simulink model "Copy_of_AB_Final_of_MPC_Bandwidth_Result"  (R2022b)
settings: Solver=FixedStepDiscrete  StartTime=0.0  StopTime=Inf  FixedStep=100e-6  RelTol=1e-3  EnableMultiTasking=on
undefined symbols (not defined in the file): C28x, CPU1, CPU2, CurrentBypassValue, DiscIntNeverNeededParam, Down, GPTRIP1SEL, TZ1, Up
libraries: c2802xlib x31, simulink x22, dspstat3 x17, dspsigops x9, c2837xDlib x6, c280xlib x5, PID_Lib x2, c2000lib x1, spsAlphaBetaZerotoabcLib x1, spsAlphaBetaZerotodq0Lib x1
(part 1 of 8)
settings Model: ExtModeTrigDuration=8  Creator=user  LastModifiedBy=user
settings SolverCC: AutoInsertRateTranBlk=on
settings OptimizationCC: DefaultParameterBehavior=Inlined  DefaultUnderspecifiedDataType=single  EnhancedBackFolding=on  PassReuseOutputArgsAs=Individual arguments  MaxStackSize=1024  OptimizeBlockOrder=speed  DifferentSizesBufferReuse=on  OptimizationCustomize=off  DenormalBehavior=FlushToZero  EfficientTunableParamExpr=on
settings DebuggingCC: ParameterTunabilityLossMsg=error
settings HardwareCC: ProdBitPerChar=16  ProdBitPerInt=16  ProdBitPerPointer=32  ProdBitPerSizeT=32  ProdBitPerPtrDiffT=32  ProdLargestAtomicInteger=Integer  ProdLargestAtomicFloat=None  ProdWordSize=16  ProdLongLongMode=on  ProdHWDeviceType=Texas Instruments->C2000
settings ModelReferenceCC: ModelReferenceNumInstancesAllowed=Single
settings SFSimCC: MATLABDynamicMemAlloc=off
settings RTWCC: Description=Embedded Coder  SystemTargetFile=ert.tlc  HardwareBoard=TI Delfino F28379D LaunchPad  TLCOptions=-aInlineSetEventsForThisBaseRateFcn=TLC_FALSE -aSuppressMultiTaskScheduler=TLC_FALSE -aRateBasedStepFcn=1  TemplateMakefile=ert_default_tmf  GenerateReport=on  Toolchain=Texas Instruments Code Composer Studio (C2000)  LaunchReport=on
settings CodeAppCC: ForceParamTrailComments=on  IgnoreCustomStorageClasses=off  OperatorAnnotations=on  SimulinkDataObjDesc=on  SFDataObjDesc=on  InsertBlockDesc=on
settings ERTTargetCC: CodeReplacementLibrary=TI C28x  ExtModeTransport=4  ExtModeStaticAlloc=on  ExtModeAutomaticAllocSize=off  ExtModeStaticAllocSize=10000  ExtModeMexFile=ext_xcp  ExtModeIntrfLevel=Level2 - Open  InlinedParameterPlacement=NonHierarchical

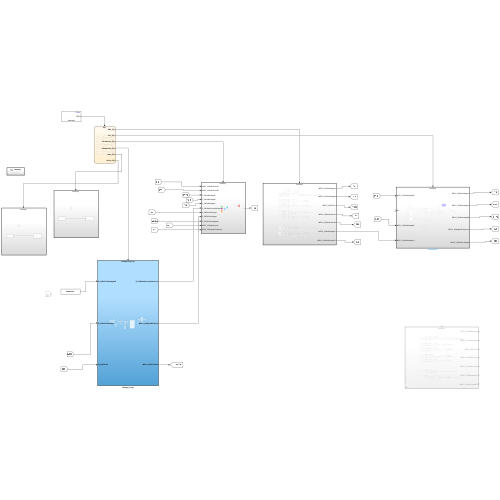
[thumbnail: Simulink's stored preview of the top-level diagram]
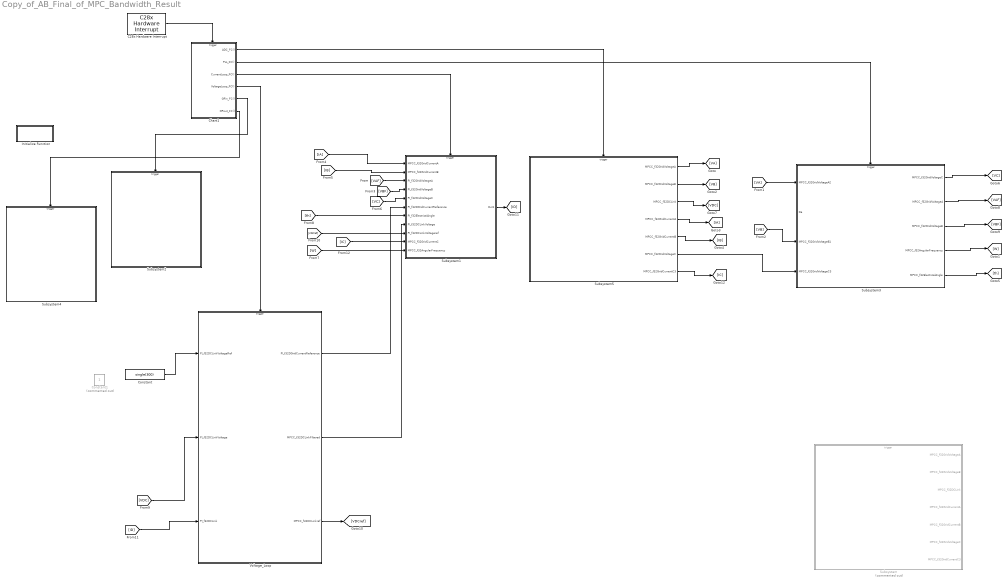
== system Copy_of_AB_Final_of_MPC_Bandwidth_Result ==
  C28x Hardware Interrupt : c2000lib/Scheduling/C28x Hardware Interrupt  irqnumbers=[1]  pienumbers=[1]  irqpriorities=[1]  irqpreempts=[0]  showinput=off  dspchiptype=C280X
  Chart1 : Stateflow chart  TreatAsAtomicUnit=on
  Constant : Constant  Value=single(300)
  Constant1 : Constant  Commented=on
  Initialize Function : Subsystem  TreatAsAtomicUnit=on
  Subsystem : Subsystem  Commented=on
  Subsystem1 : Subsystem
  Subsystem2 : Subsystem
  Subsystem3 : Subsystem
  Subsystem4 : Subsystem
  Subsystem5 : Subsystem
  Voltage_Loop : Subsystem
  wires:
  Chart1/5(GPin_FC()) -> Subsystem2/Trigger
  Chart1/3(CurrentLoop_FC()) -> Subsystem1/Trigger
  Chart1/4(VoltageLoop_FC()) -> Voltage_Loop/Trigger
  C28x Hardware Interrupt/1 -> Chart1/Trigger
  Chart1/6(GPout_FC()) -> Subsystem4/Trigger
  Chart1/2(PLL_FC()) -> Subsystem3/Trigger
  Chart1/1(ADC_FC()) -> Subsystem5/Trigger
  [IA] -> Subsystem1/1(MPCC_f32GridCurrentA)
  [IB] -> Subsystem1/2(MPCC_f32GridCurrentB)
  Subsystem3/1(MPCC_f32GridVoltageC) -> [VC]
  [th] -> Subsystem1/7(PI_f32ElectricalAngle)
  Voltage_Loop/2(MPCC_f32DCLinkFiltered) -> Subsystem1/8(PI_f32DCLinkVoltage)
  Voltage_Loop/1(PI_f32DGridCurrentReference) -> Subsystem1/6(PI_f32DGridCurrentReference)
  [VA] -> Subsystem3/1(MPCC_f32GridVoltageA2)
  [VAF] -> Subsystem1/3(PI_f32GridVoltageA)
  [VC] -> Subsystem1/5(PI_f32GridVoltageC)
  [VBF] -> Subsystem1/4(PI_f32GridVoltageB)
  Subsystem3/2(MPCC_f32GridVoltageA) -> [VAF]
  Subsystem3/3(MPCC_f32GridVoltageB) -> [VBF]
  Voltage_Loop/3(MPCC_f32DCLinkref) -> [VDCref]
  [VDCref] -> Subsystem1/9(PI_f32DCLinkVoltageref)
  [VDC] -> Voltage_Loop/2(PI_f32DCLinkVoltage)
  Constant/1 -> Voltage_Loop/1(PI_f32DCLinkVoltageRef)
  [VB] -> Subsystem3/3(MPCC_f32GridVoltageB1)
  Subsystem1/1(Out1) -> [ID]
  [ID] -> Voltage_Loop/3(PI_f32DCLink)
  [IC] -> Subsystem1/10(MPCC_f32GridCurrentC)
  [W] -> Subsystem1/11(MPCC_f32AngularFrequency)
  Subsystem3/4(MPCC_f32AngularFrequency) -> [W]
  Subsystem3/5(MPCC_f32ElectricalAngle) -> [th]
  Subsystem5/2(MPCC_f32GridVoltageB) -> [VB]
  Subsystem5/1(MPCC_f32GridVoltageA) -> [VA]
  Subsystem5/3(MPCC_f32DCLink) -> [VDC]
  Subsystem5/4(MPCC_f32GridCurrentA) -> [IA]
  Subsystem5/5(MPCC_f32GridCurrentB) -> [IB]
  Subsystem5/7(MPCC_f32GridCurrentC3) -> [IC]
  Subsystem5/6(MPCC_f32GridVoltageC) -> Subsystem3/4(MPCC_f32GridVoltageC3)

== system Copy_of_AB_Final_of_MPC_Bandwidth_Result/Initialize Function ==
  Constant : Constant  Value=boolean(0)
  Digital Output : c2837xDlib/Digital Output  GPIO_Number=GPIO8~GPIO15  GPIO_Bit0=off  GPIO_BIT0_Toggle=off  GPIO_Bit1=off  GPIO_BIT1_Toggle=off  GPIO_Bit2=off  GPIO_BIT2_Toggle=off  GPIO_Bit3=on  GPIO_BIT3_Toggle=off  GPIO_Bit4=off  GPIO_BIT4_Toggle=off  GPIO_Bit5=off  GPIO_BIT5_Toggle=off  GPIO_Bit6=off  GPIO_BIT6_Toggle=off  GPIO_Bit7=off  GPIO_BIT7_Toggle=off
  Event Listener : EventListener  DisableCoverage=on  EventName=reset
  wires:
  Constant/1 -> Digital Output/1

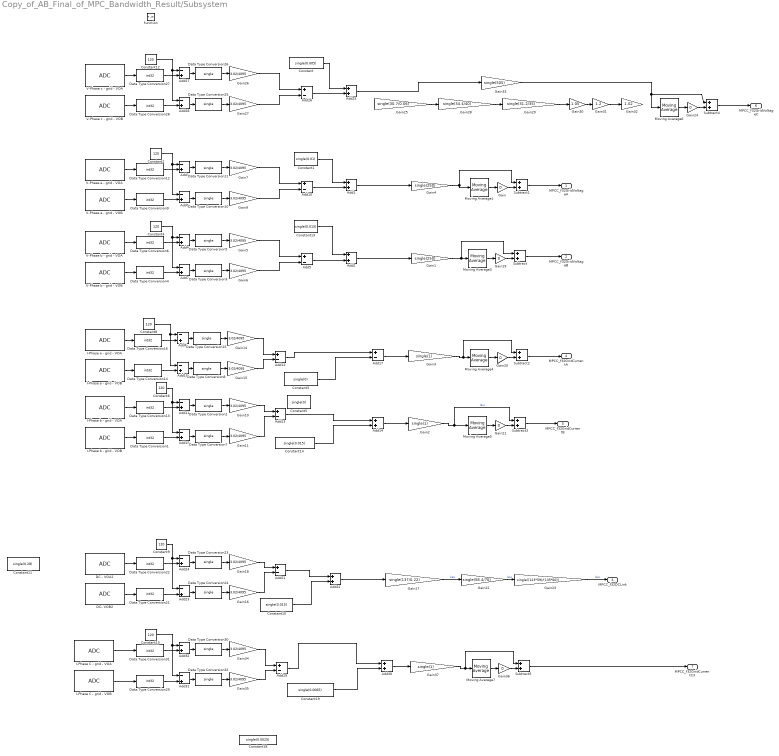
== system Copy_of_AB_Final_of_MPC_Bandwidth_Result/Subsystem ==
  function : TriggerPort  TriggerType=function-call  VariantControl=(inherit)
  Add{1..2,14,22,25,30} (6 alike) : Sum  AccumDataTypeStr=single  OutDataTypeStr=single
  Add{5,10,12..13,17,21,26,29} (8 alike) : Sum  Inputs=+-  AccumDataTypeStr=single  OutDataTypeStr=single
  Add{3..4,6..7,9,11,15,18,23..24,27..28,31..32} (14 alike) : Sum  Inputs=-+  AccumDataTypeStr=single  OutDataTypeStr=single
  Constant : Constant  Value=single(0.005)
  Constant1 : Constant  Value=single(0.01)
  Constant10 : Constant  Value=single(0.015)
  Constant11 : Constant  Value=single(0.28)
  Constant{2,4,6,8..9,12,15} (7 alike) : Constant  Value=120  OutDataTypeStr=single
  Constant13 : Constant  Value=single(0.015)
  Constant14 : Constant  Value=single(0.015)
  Constant18 : Constant  Value=single(0.0025)
  Constant19 : Constant  Value=single(0.0065)
  Constant3 : Constant  Value=single(0)
  Constant5 : Constant  Value=single(0)
  DC - VOA2 : c2802xlib/ADC  blkParamProc=C2000_Type4  ADCModule=C  samplingMode=Single sample mode  ADCResolution=12-bit (Single-ended input)  useSOC1=SOC0  useSOC2=SOC0_SOC1  SOCAcquisitionWindow=22  SOCTriggerSource=ePWM1_ADCSOCA  SOCInterruptTrigger=No ADCINT  Ts=-1  dType=uint16  postInterrupt=off  interruptSel=ADCINT1  ADCINTContinuous=on  endma=off  chdma=1  conv1=ADCINA0  conv2=ADCINA0 and ADCINB0  conv1_Type4=ADCIN5  conv2_Type4=ADCIN0 and ADCIN1
  DC- VOB2 : c2802xlib/ADC  blkParamProc=C2000_Type4  ADCModule=B  samplingMode=Single sample mode  ADCResolution=12-bit (Single-ended input)  useSOC1=SOC3  useSOC2=SOC0_SOC1  SOCAcquisitionWindow=22  SOCTriggerSource=ePWM1_ADCSOCA  SOCInterruptTrigger=No ADCINT  Ts=-1  dType=uint16  postInterrupt=off  interruptSel=ADCINT2  ADCINTContinuous=on  endma=off  chdma=1  conv1=ADCINA0  conv2=ADCINA0 and ADCINB0  conv1_Type4=ADCIN5  conv2_Type4=ADCIN2 and ADCIN3
  Data Type Conversion{1,4,6,9,12..14,16,21..22,27..29,31} (14 alike) : DataTypeConversion  OutDataTypeStr=int32  ConvertRealWorld=Stored Integer (SI)  SaturateOnIntegerOverflow=off  RndMeth=Floor
  Data Type Conversion{2..3,5,7..8,10..11,15,23..26,30,32} (14 alike) : DataTypeConversion  OutDataTypeStr=single  SaturateOnIntegerOverflow=off  RndMeth=Floor
  Gain{,19..21,24,36} (6 alike) : Gain  Gain=0
  Gain1 : Gain  Gain=single(250)
  Gain{5..7,9..11,14..16,18,26..27,34..35} (14 alike) : Gain  Gain=3.02/4095  ParamDataTypeStr=single  OutDataTypeStr=single
  Gain17 : Gain  Gain=single(137/0.22)
  Gain2 : Gain  Gain=single(1)
  Gain22 : Gain  Gain=single(58.4/70)
  Gain23 : Gain  Gain=single((123*59)/(135*60))
  Gain25 : Gain  Gain=single(30.7/0.06)
  Gain28 : Gain  Gain=single(34.4/40)
  Gain29 : Gain  Gain=single(31.2/35)
  Gain3 : Gain  Gain=single(1)
  Gain30 : Gain  Gain=1.05
  Gain31 : Gain  Gain=1.2
  Gain32 : Gain  Gain=1.02
  Gain33 : Gain  Gain=single(505)
  Gain37 : Gain  Gain=single(1)
  Gain4 : Gain  Gain=single(250)
  I-Phase C - grid - VOA : c2802xlib/ADC  blkParamProc=C2000_Type4  ADCModule=A  samplingMode=Single sample mode  ADCResolution=12-bit (Single-ended input)  useSOC1=SOC15  useSOC2=SOC0_SOC1  SOCAcquisitionWindow=22  SOCTriggerSource=ePWM1_ADCSOCA  SOCInterruptTrigger=No ADCINT  Ts=-1  dType=uint16  postInterrupt=off  interruptSel=ADCINT1  ADCINTContinuous=on  endma=off  chdma=1  conv1=ADCINA0  conv2=ADCINA0 and ADCINB0  conv1_Type4=ADCIN15  conv2_Type4=ADCIN0 and ADCIN1
  I-Phase C - grid - VOB : c2802xlib/ADC  blkParamProc=C2000_Type4  ADCModule=A  samplingMode=Single sample mode  ADCResolution=12-bit (Single-ended input)  useSOC1=SOC10  useSOC2=SOC0_SOC1  SOCAcquisitionWindow=22  SOCTriggerSource=ePWM1_ADCSOCA  SOCInterruptTrigger=No ADCINT  Ts=-1  dType=uint16  postInterrupt=off  interruptSel=ADCINT2  ADCINTContinuous=on  endma=off  chdma=1  conv1=ADCINA0  conv2=ADCINA0 and ADCINB0  conv1_Type4=ADCIN14  conv2_Type4=ADCIN2 and ADCIN3
  I-Phase a - grid - VOA : c2802xlib/ADC  blkParamProc=C2000_Type4  ADCModule=A  samplingMode=Single sample mode  ADCResolution=12-bit (Single-ended input)  useSOC1=SOC0  useSOC2=SOC0_SOC1  SOCAcquisitionWindow=22  SOCTriggerSource=ePWM1_ADCSOCA  SOCInterruptTrigger=No ADCINT  Ts=-1  dType=uint16  postInterrupt=on  interruptSel=ADCINT1  ADCINTContinuous=on  endma=off  chdma=1  conv1=ADCINA0  conv2=ADCINA0 and ADCINB0  conv1_Type4=ADCIN4  conv2_Type4=ADCIN0 and ADCIN1
  I-Phase a - grid - VOB : c2802xlib/ADC  blkParamProc=C2000_Type4  ADCModule=B  samplingMode=Single sample mode  ADCResolution=12-bit (Single-ended input)  useSOC1=SOC1  useSOC2=SOC0_SOC1  SOCAcquisitionWindow=22  SOCTriggerSource=ePWM1_ADCSOCA  SOCInterruptTrigger=No ADCINT  Ts=-1  dType=uint16  postInterrupt=off  interruptSel=ADCINT2  ADCINTContinuous=on  endma=off  chdma=1  conv1=ADCINA0  conv2=ADCINA0 and ADCINB0  conv1_Type4=ADCIN4  conv2_Type4=ADCIN2 and ADCIN3
  I-Phase b - grid - VOA : c2802xlib/ADC  blkParamProc=C2000_Type4  ADCModule=C  samplingMode=Single sample mode  ADCResolution=12-bit (Single-ended input)  useSOC1=SOC12  useSOC2=SOC0_SOC1  SOCAcquisitionWindow=22  SOCTriggerSource=ePWM1_ADCSOCA  SOCInterruptTrigger=No ADCINT  Ts=-1  dType=uint16  postInterrupt=off  interruptSel=ADCINT1  ADCINTContinuous=on  endma=off  chdma=1  conv1=ADCINA0  conv2=ADCINA0 and ADCINB0  conv1_Type4=ADCIN4  conv2_Type4=ADCIN0 and ADCIN1
  I-Phase b - grid - VOB : c2802xlib/ADC  blkParamProc=C2000_Type4  ADCModule=A  samplingMode=Single sample mode  ADCResolution=12-bit (Single-ended input)  useSOC1=SOC3  useSOC2=SOC0_SOC1  SOCAcquisitionWindow=22  SOCTriggerSource=ePWM1_ADCSOCA  SOCInterruptTrigger=No ADCINT  Ts=-1  dType=uint16  postInterrupt=off  interruptSel=ADCINT2  ADCINTContinuous=on  endma=off  chdma=1  conv1=ADCINA0  conv2=ADCINA0 and ADCINB0  conv1_Type4=ADCIN5  conv2_Type4=ADCIN2 and ADCIN3
  Moving Average{1,3..7} (6 alike) : dspstat3/Moving Average  Method=Exponential weighting  ForgettingFactorPort=off  SpecifyWindowLength=on  WindowLength=4  OverlapLength=3  AllowArbitraryInputLength=off  ForgettingFactor=0.99  SimulateUsing=Code generation
  Subtract{,1..5} (6 alike) : Sum
  V-Phase a - grid - VOA : c2802xlib/ADC  blkParamProc=C2000_Type4  ADCModule=C  samplingMode=Single sample mode  ADCResolution=12-bit (Single-ended input)  useSOC1=SOC4  useSOC2=SOC0_SOC1  SOCAcquisitionWindow=22  SOCTriggerSource=ePWM1_ADCSOCA  SOCInterruptTrigger=No ADCINT  Ts=-1  dType=uint16  postInterrupt=off  interruptSel=ADCINT1  ADCINTContinuous=on  endma=off  chdma=1  conv1=ADCINA0  conv2=ADCINA0 and ADCINB0  conv1_Type4=ADCIN3  conv2_Type4=ADCIN0 and ADCIN1
  V-Phase a - grid - VOB : c2802xlib/ADC  blkParamProc=C2000_Type4  ADCModule=B  samplingMode=Single sample mode  ADCResolution=12-bit (Single-ended input)  useSOC1=SOC5  useSOC2=SOC0_SOC1  SOCAcquisitionWindow=22  SOCTriggerSource=ePWM1_ADCSOCA  SOCInterruptTrigger=No ADCINT  Ts=-1  dType=uint16  postInterrupt=off  interruptSel=ADCINT2  ADCINTContinuous=on  endma=off  chdma=1  conv1=ADCINA0  conv2=ADCINA0 and ADCINB0  conv1_Type4=ADCIN3  conv2_Type4=ADCIN2 and ADCIN3
  V-Phase b - grid - VOA : c2802xlib/ADC  blkParamProc=C2000_Type4  ADCModule=A  samplingMode=Single sample mode  ADCResolution=12-bit (Single-ended input)  useSOC1=SOC6  useSOC2=SOC0_SOC1  SOCAcquisitionWindow=22  SOCTriggerSource=ePWM1_ADCSOCA  SOCInterruptTrigger=No ADCINT  Ts=-1  dType=uint16  postInterrupt=off  interruptSel=ADCINT1  ADCINTContinuous=on  endma=off  chdma=1  conv1=ADCINA0  conv2=ADCINA0 and ADCINB0  conv1_Type4=ADCIN3  conv2_Type4=ADCIN0 and ADCIN1
  V-Phase b - grid - VOB : c2802xlib/ADC  blkParamProc=C2000_Type4  ADCModule=C  samplingMode=Single sample mode  ADCResolution=12-bit (Single-ended input)  useSOC1=SOC7  useSOC2=SOC0_SOC1  SOCAcquisitionWindow=22  SOCTriggerSource=ePWM1_ADCSOCA  SOCInterruptTrigger=No ADCINT  Ts=-1  dType=uint16  postInterrupt=off  interruptSel=ADCINT2  ADCINTContinuous=on  endma=off  chdma=1  conv1=ADCINA0  conv2=ADCINA0 and ADCINB0  conv1_Type4=ADCIN2  conv2_Type4=ADCIN2 and ADCIN3
  V-Phase c - grid - VOA : c2802xlib/ADC  blkParamProc=C2000_Type4  ADCModule=B  samplingMode=Single sample mode  ADCResolution=12-bit (Single-ended input)  useSOC1=SOC0  useSOC2=SOC0_SOC1  SOCAcquisitionWindow=22  SOCTriggerSource=ePWM1_ADCSOCA  SOCInterruptTrigger=No ADCINT  Ts=-1  dType=uint16  postInterrupt=off  interruptSel=ADCINT1  ADCINTContinuous=on  endma=off  chdma=1  conv1=ADCINA0  conv2=ADCINA0 and ADCINB0  conv1_Type4=ADCIN2  conv2_Type4=ADCIN0 and ADCIN1
  V-Phase c - grid - VOB : c2802xlib/ADC  blkParamProc=C2000_Type4  ADCModule=A  samplingMode=Single sample mode  ADCResolution=12-bit (Single-ended input)  useSOC1=SOC1  useSOC2=SOC0_SOC1  SOCAcquisitionWindow=22  SOCTriggerSource=ePWM1_ADCSOCA  SOCInterruptTrigger=No ADCINT  Ts=-1  dType=uint16  postInterrupt=off  interruptSel=ADCINT2  ADCINTContinuous=on  endma=off  chdma=1  conv1=ADCINA0  conv2=ADCINA0 and ADCINB0  conv1_Type4=ADCIN2  conv2_Type4=ADCIN2 and ADCIN3
  MPCC_f32GridVoltageA : Outport
  MPCC_f32GridVoltageB : Outport  Port=2
  MPCC_f32DCLink : Outport  Port=3
  MPCC_f32GridCurrentA : Outport  Port=4
  MPCC_f32GridCurrentB : Outport  Port=5
  MPCC_f32GridVoltageC : Outport  Port=6
  MPCC_f32GridCurrentC3 : Outport  Port=7
  wires:
  Gain5/1 -> Add5/1
  Data Type Conversion5/1 -> Gain5/1
  Gain1/1 -> Subtract/1, Moving Average3/1
  Add9/1 -> Data Type Conversion10/1
  V-Phase a - grid - VOB/1 -> Data Type Conversion9/1
  Data Type Conversion9/1 -> Add9/2
  Gain7/1 -> Add10/1
  Data Type Conversion10/1 -> Gain9/1
  Data Type Conversion12/1 -> Add3/2
  Add7/1 -> Data Type Conversion3/1
  Data Type Conversion4/1 -> Add7/2
  Data Type Conversion6/1 -> Add4/2
  Gain9/1 -> Add10/2
  V-Phase b - grid - VOB/1 -> Data Type Conversion4/1
  V-Phase b - grid - VOA/1 -> Data Type Conversion6/1
  Add4/1 -> Data Type Conversion5/1
  Add3/1 -> Data Type Conversion11/1
  Data Type Conversion3/1 -> Gain6/1
  Gain6/1 -> Add5/2
  Constant4/1 -> Add7/1, Add4/1
  V-Phase a - grid - VOA/1 -> Data Type Conversion12/1
  Constant2/1 -> Add9/1, Add3/1
  Data Type Conversion11/1 -> Gain7/1
  Add10/1 -> Add1/2
  Add5/1 -> Add2/2
  Add1/1 -> Gain4/1
  Add2/1 -> Gain1/1
  I-Phase b - grid - VOA/1 -> Data Type Conversion13/1
  Data Type Conversion15/1 -> Gain14/1
  Data Type Conversion8/1 -> Gain15/1
  Data Type Conversion14/1 -> Add18/2
  Gain15/1 -> Add12/2
  Data Type Conversion13/1 -> Add11/2
  Data Type Conversion16/1 -> Add6/2
  Gain14/1 -> Add12/1
  Add6/1 -> Data Type Conversion15/1
  Gain10/1 -> Add13/1
  Add18/1 -> Data Type Conversion8/1
  I-Phase a - grid - VOA/1 -> Data Type Conversion16/1
  Gain2/1 -> Subtract3/1, Moving Average5/1  "Iau"
  Add12/1 -> Add17/1
  Add13/1 -> Add14/1
  Data Type Conversion2/1 -> Gain10/1
  Constant6/1 -> Add15/1, Add11/1
  I-Phase b - grid - VOB/1 -> Data Type Conversion1/1
  Data Type Conversion1/1 -> Add15/2
  Gain11/1 -> Add13/2
  Add17/1 -> Gain3/1
  Add11/1 -> Data Type Conversion2/1
  Add14/1 -> Gain2/1
  Constant8/1 -> Add18/1, Add6/1
  I-Phase a - grid - VOB/1 -> Data Type Conversion14/1
  Data Type Conversion7/1 -> Gain11/1
  Add15/1 -> Data Type Conversion7/1
  Subtract/1 -> MPCC_f32GridVoltageB/1
  Moving Average3/1 -> Gain19/1
  Moving Average1/1 -> Gain/1
  Gain4/1 -> Subtract1/1, Moving Average1/1
  Subtract1/1 -> MPCC_f32GridVoltageA/1
  Moving Average4/1 -> Gain20/1
  Gain3/1 -> Subtract2/1, Moving Average4/1
  Moving Average5/1 -> Gain21/1
  Data Type Conversion22/1 -> Add24/2
  DC- VOB2/1 -> Data Type Conversion21/1
  Data Type Conversion21/1 -> Add23/2
  Data Type Conversion23/1 -> Gain18/1
  DC - VOA2/1 -> Data Type Conversion22/1
  Add24/1 -> Data Type Conversion23/1
  Constant9/1 -> Add23/1, Add24/1
  Gain16/1 -> Add21/2
  Add23/1 -> Data Type Conversion24/1
  Data Type Conversion24/1 -> Gain16/1
  Gain18/1 -> Add21/1
  Gain/1 -> Subtract1/2
  Gain19/1 -> Subtract/2
  Gain20/1 -> Subtract2/2
  Gain21/1 -> Subtract3/2
  Gain17/1 -> Gain22/1  "Iau"
  Subtract2/1 -> MPCC_f32GridCurrentA/1
  Subtract3/1 -> MPCC_f32GridCurrentB/1
  Constant10/1 -> Add22/2
  Gain22/1 -> Gain23/1  "Iau"
  Constant13/1 -> Add2/1
  Constant1/1 -> Add1/1
  Gain23/1 -> MPCC_f32DCLink/1  "Iau"
  V-Phase c - grid - VOB/1 -> Data Type Conversion28/1
  Gain26/1 -> Add26/1
  Data Type Conversion25/1 -> Gain27/1
  V-Phase c - grid - VOA/1 -> Data Type Conversion27/1
  Subtract4/1 -> MPCC_f32GridVoltageC/1
  Add26/1 -> Add25/2
  Data Type Conversion26/1 -> Gain26/1
  Data Type Conversion27/1 -> Add27/2
  Moving Average6/1 -> Gain24/1
  Data Type Conversion28/1 -> Add28/2
  Gain27/1 -> Add26/2
  Add28/1 -> Data Type Conversion25/1
  Constant12/1 -> Add28/1, Add27/1
  Add27/1 -> Data Type Conversion26/1
  Gain25/1 -> Gain28/1
  Constant/1 -> Add25/1
  Gain24/1 -> Subtract4/2
  Gain28/1 -> Gain29/1
  Gain29/1 -> Gain30/1
  Gain30/1 -> Gain31/1
  Gain31/1 -> Gain32/1
  Add25/1 -> Gain33/1
  Gain33/1 -> Subtract4/1, Moving Average6/1
  Add31/1 -> Data Type Conversion32/1
  Data Type Conversion32/1 -> Gain35/1
  Data Type Conversion31/1 -> Add32/2
  Gain34/1 -> Add29/1
  Constant15/1 -> Add31/1, Add32/1
  Gain35/1 -> Add29/2
  Subtract5/1 -> MPCC_f32GridCurrentC3/1
  Gain36/1 -> Subtract5/2
  Data Type Conversion30/1 -> Gain34/1
  Constant19/1 -> Add30/2
  Add29/1 -> Add30/1
  Data Type Conversion29/1 -> Add31/2
  I-Phase C - grid - VOB/1 -> Data Type Conversion29/1
  I-Phase C - grid - VOA/1 -> Data Type Conversion31/1
  Gain37/1 -> Subtract5/1, Moving Average7/1
  Add32/1 -> Data Type Conversion30/1
  Add30/1 -> Gain37/1
  Moving Average7/1 -> Gain36/1
  Add22/1 -> Gain17/1
  Add21/1 -> Add22/1
  Constant14/1 -> Add14/2
  Constant3/1 -> Add17/2

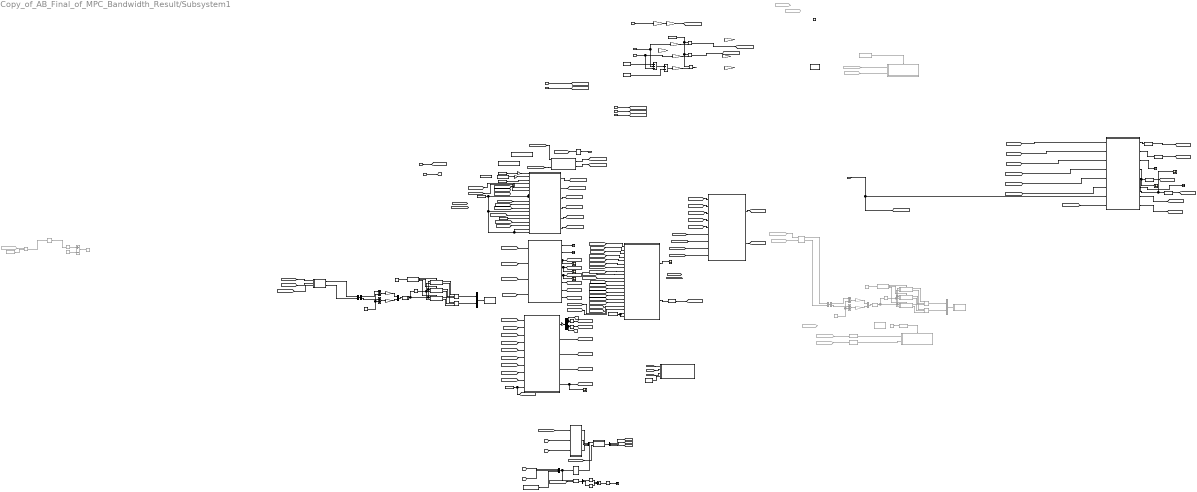
== system Copy_of_AB_Final_of_MPC_Bandwidth_Result/Subsystem1 ==
  MPCC_f32GridCurrentA : Inport
  MPCC_f32GridCurrentB : Inport  Port=2
  PI_f32GridVoltageA : Inport  Port=3
  PI_f32GridVoltageB : Inport  Port=4
  PI_f32GridVoltageC : Inport  Port=5
  PI_f32DGridCurrentReference : Inport  Port=6
  PI_f32ElectricalAngle : Inport  Port=7
  PI_f32DCLinkVoltage : Inport  Port=8
  PI_f32DCLinkVoltageref : Inport  Port=9
  MPCC_f32GridCurrentC : Inport  Port=10
  MPCC_f32AngularFrequency : Inport  Port=11
  function : TriggerPort  TriggerType=function-call  VariantControl=(inherit)
  ABCtoDQO : Subsystem
  Add : Sum  Commented=on
  Add1 : Sum  Inputs=+--
  Add10 : Sum
  Add2 : Sum  Inputs=+-
  Add3 : Sum  Commented=on
  Add4 : Sum
  Add5 : Sum
  Alpha-Beta-Zero to abc : spsAlphaBetaZerotoabcLib/Alpha-Beta-Zero to abc
      settings: LibrarySourceBlock=|
      | sps_lib/Control/Alpha-Beta-Zero
      | to abc
  Alpha-Beta-Zero to dq0 : spsAlphaBetaZerotodq0Lib/Alpha-Beta-Zero to dq0  Alignment=Aligned with phase A axis
  AlphaBetaDutiesCalculation : Subsystem
  AlphaBetaVoltageReferenceCalculation : Subsystem
  Bus Creator : BusCreator  Commented=on  Inputs=2
  Bus Creator1 : BusCreator  Inputs=2
  Bus Selector1 : BusSelector  Commented=on  OutputSignals=signal1,signal2
  Bus Selector2 : BusSelector  OutputSignals=signal1,signal2
  Cast To Boolean : DataTypeConversion  Commented=on  OutDataTypeStr=boolean  SaturateOnIntegerOverflow=off  RndMeth=Floor
  Cast To Single{,1..3,6} (5 alike) : DataTypeConversion  OutDataTypeStr=single  SaturateOnIntegerOverflow=off  RndMeth=Floor
  Cast To Single10 : DataTypeConversion  Commented=on  OutDataTypeStr=single  SaturateOnIntegerOverflow=off  RndMeth=Floor
  Cast To Single9 : DataTypeConversion  Commented=on  OutDataTypeStr=single  SaturateOnIntegerOverflow=off  RndMeth=Floor
  CodeGeneration : Subsystem  Commented=on  TreatAsAtomicUnit=on
  CodeGeneration1 : Subsystem  TreatAsAtomicUnit=on
  Constant{1,10..11,19,48} (5 alike) : Constant  Value=single(0)
  Constant16 : Constant  Value=10  OutDataTypeStr=single
  Constant18 : Constant  Value=single(9.5e-3)
  Constant2 : Constant  Value=single(0.005)
  Constant20 : Constant  Value=single(0.34)
  Constant21 : Constant  Value=single(18.5825e-3)
  Constant22 : Constant  Value=single(100e-6)
  Constant25 : Constant  Value=boolean(0)
  Constant26 : Constant  Value=single(1/10000)
  Constant3 : Constant  Commented=on  Value=10  OutDataTypeStr=single
  Constant30 : Constant  Commented=on  Value=single(sqrt(3))
  Constant36 : Constant  Commented=on
  Constant37 : Constant  Commented=on  Value=boolean(1)
  Constant51 : Constant  Value=single(1)
  Counter Limited : simulink/Sources/Counter Limited  Commented=on  uplimit=599  tsamp=-1
  Counter Limited1 : simulink/Sources/Counter Limited  uplimit=599  tsamp=-1
  Data : Subsystem  Commented=on  TreatAsAtomicUnit=on
  Data1 : Subsystem  TreatAsAtomicUnit=on
  Data_Conditioning : Subsystem  Commented=on
  Data_Conditioning1 : Subsystem
  Delay : Delay  DelayLength=1  InitialCondition=200
  Delay1 : Delay  DelayLength=1  InitialCondition=-200
  Demux : Demux  Outputs=2
  Demux1 : Demux  Outputs=3
  Demux2 : Demux  Outputs=3
  Digital Input : c280xlib/Digital Input  Commented=on  GPIO_Number=GPIO32~GPIO34  GPIO_Bit0=on  GPIO_Bit1=off  GPIO_Bit2=off  GPIO_Bit3=off  GPIO_Bit4=off  GPIO_Bit5=off  GPIO_Bit6=off  GPIO_Bit7=off  sampleTime=-1  dataType=boolean  GPIO_Bit0_Qualification=Sync to SYSCLKOUT  GPIO_Bit1_Qualification=Sync to SYSCLKOUT  GPIO_Bit2_Qualification=Sync to SYSCLKOUT  GPIO_Bit3_Qualification=Sync to SYSCLKOUT  GPIO_Bit4_Qualification=Sync to SYSCLKOUT  GPIO_Bit5_Qualification=Sync to SYSCLKOUT  GPIO_Bit6_Qualification=Sync to SYSCLKOUT  GPIO_Bit7_Qualification=Sync to SYSCLKOUT  Qualification_Period=-1
  Divide4 : Product  Commented=on  Inputs=*/  RndMeth=Zero  SaturateOnIntegerOverflow=on
  End : Subsystem  Commented=on  TreatAsAtomicUnit=on
  End1 : Subsystem  TreatAsAtomicUnit=on
  From10 : From  Commented=on  GotoTag=MPCC_f32AngularFrequency
  From103 : From  Commented=on  GotoTag=PI_f32DCLinkVoltage
  From106 : From  Commented=on  GotoTag=PI_f32QGridCurrent
  From123 : From  Commented=on  GotoTag=PI_f32GridVoltageA
  From124 : From  Commented=on  GotoTag=MPCC_f32ElectricalAngle
  From128 : From  Commented=on  GotoTag=PI_f32DGridCurrentReference
  From129 : From  Commented=on  GotoTag=PI_f32DGridCurrent
  From16 : From  Commented=on  GotoTag=PI_f32DCLinkVoltageref
  From18 : From  Commented=on  GotoTag=PI_f32QGridCurrent
  From7 : From  Commented=on  GotoTag=PI_f32DGridCurrent
  Gain : Gain  Gain=single(-1)
  Gain1 : Gain  Gain=single(-1)
  Gain10 : Gain  Gain=1000  OutDataTypeStr=single
  Gain11 : Gain  Gain=1.5
  Gain12 : Gain  Gain=1.5
  Gain2 : Gain  Gain=single(6.25)
  Gain20 : Gain  Gain=single(5.85)
  Gain21 : Gain  Gain=single(1)
  Gain23 : Gain  Gain=-1
  Gain3 : Gain  Gain=single(5.94)
  Gain4 : Gain  Gain=single(5.94)
  Gain5 : Gain  Gain=single(-1)
  Gain6 : Gain  Commented=on  Gain=1000  OutDataTypeStr=single
  Gain7 : Gain  Commented=on  Gain=1000  OutDataTypeStr=single
  Gain8 : Gain  Gain=1000  OutDataTypeStr=single
  Gain9 : Gain  Gain=single(5.94)
  GridCurrentFirstPrediction : Subsystem
  GridCurrentSecondPrediction : Subsystem
  If : If  Commented=on  IfExpression=u1 == 0  ElseIfExpressions=u1 == 599
  If1 : If  IfExpression=u1 == 0  ElseIfExpressions=u1 == 599
  Merge : Merge  Commented=on  Inputs=3
  Merge1 : Merge  Commented=on  Inputs=3
  Merge2 : Merge  Inputs=3
  Merge3 : Merge  Inputs=3
  ModulatorTimes : Subsystem
  Mux : Mux  Commented=on  Inputs=2
  Mux1 : Mux  Commented=on  Inputs=2
  Mux2 : Mux  Inputs=2
  Mux3 : Mux  Inputs=2
  Mux4 : Mux  Inputs=3
  Mux6 : Mux  Inputs=3
  Product : Product
  Product1 : Product
  Product2 : Product
  SOGI 1st : Subsystem  Commented=on
  SVM : Subsystem
  Scope{,1..6} (7 alike) : Scope
  Signal Copy : SignalConversion  Commented=on  OverrideOpt=off
  Signal Copy1 : SignalConversion  OverrideOpt=off
  Sqrt : Sqrt  Commented=on
  Sqrt1 : Sqrt
  Square : Math  Commented=on  Operator=square
  Square1 : Math  Commented=on  Operator=square
  Square2 : Math  Operator=square
  Square3 : Math  Operator=square
  Start : Subsystem  Commented=on  TreatAsAtomicUnit=on
  Start1 : Subsystem  TreatAsAtomicUnit=on
  Subsystem : Subsystem
  Subsystem1 : Subsystem  Commented=on
  Subsystem2 : Subsystem  Commented=on
  Subsystem6 : Subsystem
  Subtract : Sum  Commented=on  Inputs=+-
  System Outputs : Subsystem  mask(System Outputs){ShowInLibBrowser=0}
      mask prompts: ShowInLibBrowser "Simulink:masks:CustCodeMaskParam1_MP"
      settings: CopyFcn=cccopyfcn(gcb)  OpenFcn=ccopenfcn('System Outputs Function')
      mask Help: eval('feval(''rtwprivate'',''rtwhelpview'',''rtw_sys_outputs_block'')');
      mask Display: disp('System\nOutputs');
  Terminator{,6..7,10..11} (5 alike) : Terminator
  VoltageReferenceCalculation : Subsystem
  Width : Width  Commented=on  OutDataTypeMode=All ports same datatype  DataType=uint16
  Width1 : Width  OutDataTypeMode=All ports same datatype  DataType=uint16
  dq_abc1 : Subsystem
  nominal : Constant  Value=single(0.7)  VectorParams1D=off  SampleTime=-1
  underload : Constant  Value=single(0.1)  VectorParams1D=off  SampleTime=-1
  Out1 : Outport
  wires:
  Add1/1 -> Add2/1
  Constant2/1 -> Add2/2
  Add2/1 -> Gain4/1
  MPCC_f32GridCurrentA/1 -> Gain2/1, Add1/2
  MPCC_f32GridCurrentB/1 -> Add1/3, Gain3/1
  Constant1/1 -> Add1/1
  [PI_f32GridCurrentA] -> ABCtoDQO/1(PI_f32GridCurrentA)
  ABCtoDQO/6(PI_f32OGridVoltage) -> Terminator6/1
  [PI_f32GridVoltageB] -> ABCtoDQO/5(PI_f32GridVoltageB)
  ABCtoDQO/1(PI_f32DGridCurrent) -> Cast To Single1/1
  [PI_f32GridVoltageC] -> ABCtoDQO/6(PI_f32GridVoltageC)
  ABCtoDQO/5(PI_f32QGridVoltage) -> Scope4/1, Cast To Single3/1
  [PI_f32GridCurrentB] -> ABCtoDQO/2(PI_f32GridCurrentB)
  [PI_f32GridCurrentC] -> ABCtoDQO/3(PI_f32GridCurrentC)
  ABCtoDQO/3(PI_f32OGridCurrent) -> Terminator7/1
  ABCtoDQO/2(PI_f32QGridCurrent) -> Cast To Single2/1
  ABCtoDQO/4(PI_f32DGridVoltage) -> Scope3/1, Cast To Single6/1
  PI_f32GridVoltageC/1 -> [PI_f32GridVoltageC]
  PI_f32GridVoltageB/1 -> [PI_f32GridVoltageB]
  PI_f32GridVoltageA/1 -> [PI_f32GridVoltageA]
  PI_f32ElectricalAngle/1 -> [MPCC_f32ElectricalAngle], ABCtoDQO/7(PI_f32ElectricalAngle)
  PI_f32DCLinkVoltage/1 -> [PI_f32DCLinkVoltage]
  [PI_f32GridVoltageA] -> ABCtoDQO/4(PI_f32GridVoltageA)
  ? -> ?
  VoltageReferenceCalculation/5(MPCC_f32Predictionterm_B) -> [MPCC_f32Predictionterm_B]
  [PI_f32QGridCurrentReference] -> VoltageReferenceCalculation/13(MPCC_f32QGridCurrentReference)
  Constant19/1 -> VoltageReferenceCalculation/17(MPCC_f32HarmonicDGridVoltage), VoltageReferenceCalculation/18(MPCC_f32HarmonicQGridVoltage), VoltageReferenceCalculation/12(MPCC_f32HarmonicDGridCurrentReference), VoltageReferenceCalculation/8(MPCC_f32HarmonicQGridCurrent), VoltageReferenceCalculation/7(MPCC_f32HarmonicDGridCurrent)
  VoltageReferenceCalculation/4(MPCC_f32Predictionterm_A) -> [MPCC_f32Predictionterm_A]
  Constant22/1 -> VoltageReferenceCalculation/3(MPCC_f32SamplingPeriod)
  VoltageReferenceCalculation/3(MPCC_f32ElectricalAngle_K_1) -> [MPCC_f32ElectricalAngle_K_1]
  Constant10/1 -> VoltageReferenceCalculation/14(MPCC_f32HarmonicQGridCurrentReference)
  VoltageReferenceCalculation/6(MPCC_f32Predictionterm_C) -> [MPCC_f32Predictionterm_C]
  Constant20/1 -> Gain11/1
  [MPCC_f32ElectricalAngle] -> VoltageReferenceCalculation/15(MPCC_f32ElectricalAngle)
  [PI_f32DGridCurrentReference] -> VoltageReferenceCalculation/11(MPCC_f32DGridCurrentReference)
  GridCurrentFirstPrediction/1(MPCC_f32DGridCurrent_K_1) -> [MPCC_f32DGridCurrent_K_1]
  [MPCC_f32Predictionterm_A] -> GridCurrentFirstPrediction/1(MPCC_f32Predictionterm_A)
  [MPCC_f32Predictionterm_C] -> GridCurrentFirstPrediction/3(MPCC_f32Predictionterm_C)
  [PI_f32DGridCurrent] -> GridCurrentFirstPrediction/4(MPCC_f32DGridCurrent)
  [MPCC_f32Predictionterm_B] -> GridCurrentFirstPrediction/2(MPCC_f32Predictionterm_B)
  [PI_f32QGridCurrent] -> GridCurrentFirstPrediction/5(MPCC_f32QGridCurrent)
  GridCurrentFirstPrediction/2(MPCC_f32QGridCurrent_K_1) -> [MPCC_f32QGridCurrent_K_1]
  [PI_f32DCLinkVoltage] -> AlphaBetaDutiesCalculation/4(MPCC_f32DCLinkVoltage)
  [MPCC_f32ElectricalAngle_K_1] -> AlphaBetaDutiesCalculation/3(MPCC_f32ElectricalAngle_K_1)
  AlphaBetaDutiesCalculation/3(MPCC_f32Duty_Sector1) -> Scope1/1, [MPCC_f32Duty_Sector1]
  AlphaBetaDutiesCalculation/4(MPCC_f32Duty_Sector2) -> Scope2/1, [MPCC_f32Duty_Sector2]
  [MPCC_f32DVoltageReference] -> AlphaBetaDutiesCalculation/1(MPCC_f32DVoltageReference)
  [MPCC_f32QVoltageReference] -> AlphaBetaDutiesCalculation/2(MPCC_f32QVoltageReference)
  AlphaBetaDutiesCalculation/8(MPCC_f32Duty_Sector6) -> [MPCC_f32Duty_Sector6]
  AlphaBetaDutiesCalculation/6(MPCC_f32Duty_Sector4) -> [MPCC_f32Duty_Sector4]
  AlphaBetaDutiesCalculation/2(MPCC_f32BetaVoltageReference) -> Terminator11/1
  AlphaBetaDutiesCalculation/5(MPCC_f32Duty_Sector3) -> Scope5/1, [MPCC_f32Duty_Sector3]
  AlphaBetaDutiesCalculation/7(MPCC_f32Duty_Sector5) -> [MPCC_f32Duty_Sector5]
  AlphaBetaDutiesCalculation/1(MPCC_f32AlphaVoltageReference) -> Terminator10/1
  [MPCC_f32Predictionterm_B] -> GridCurrentSecondPrediction/3(MPCC_f32Predictionterm_B)
  [PI_f32DCLinkVoltage] -> GridCurrentSecondPrediction/11(MPCC_f32DCLinkVoltage)
  [MPCC_f32Duty_Sector2] -> GridCurrentSecondPrediction/13(MPCC_f32Duty_Sector2)
  [MPCC_f32Duty_Sector6] -> GridCurrentSecondPrediction/17(MPCC_f32Duty_Sector6)
  [MPCC_f32QGridCurrent_K_1] -> GridCurrentSecondPrediction/6(MPCC_f32QGridCurrent_K_1)
  GridCurrentSecondPrediction/1(MPCC_f32MinCostFunction) -> Scope6/1
  [PI_f32QGridCurrentReference] -> GridCurrentSecondPrediction/8(MPCC_f32QGridCurrentReference)
  [MPCC_f32Duty_Sector4] -> GridCurrentSecondPrediction/15(MPCC_f32Duty_Sector4)
  [MPCC_f32Predictionterm_C] -> GridCurrentSecondPrediction/4(MPCC_f32Predictionterm_C)
  [MPCC_f32ElectricalAngle_K_1] -> GridCurrentSecondPrediction/1(MPCC_f32ElectricalAngle_K_1)
  [MPCC_f32Duty_Sector3] -> GridCurrentSecondPrediction/14(MPCC_f32Duty_Sector3)
  [PI_f32DGridCurrentReference] -> GridCurrentSecondPrediction/7(MPCC_f32DGridCurrentReference)
  [MPCC_f32Duty_Sector5] -> GridCurrentSecondPrediction/16(MPCC_f32Duty_Sector5)
  [MPCC_f32Predictionterm_A] -> GridCurrentSecondPrediction/2(MPCC_f32Predictionterm_A)
  [MPCC_f32Duty_Sector1] -> GridCurrentSecondPrediction/12(MPCC_f32Duty_Sector1)
  [MPCC_f32DGridCurrent_K_1] -> GridCurrentSecondPrediction/5(MPCC_f32DGridCurrent_K_1)
  Delay/1 -> [MPCC_f32DConvVoltage]
  ModulatorTimes/4(MPCC_f32Time0) -> [MPCC_f32Time0]
  [MPCC_f32Duty_Sector6] -> ModulatorTimes/8(MPCC_f32Duty_Sector6)
  ModulatorTimes/1(MPCC_f32DQConvVoltage) -> Gain23/1
  Constant26/1 -> [MPCC_f32SwitchingPeriod], ModulatorTimes/10(MPCC_f32SwitchingPeriod)
  ModulatorTimes/2(MPCC_f32Time1) -> [MPCC_f32Time1]
  [MPCC_f32Duty_Sector1] -> ModulatorTimes/3(MPCC_f32Duty_Sector1)
  [MPCC_f32ElectricalAngle_K_1] -> ModulatorTimes/1(MPCC_f32ElectricalAngle_K_1)
  Delay1/1 -> [MPCC_f32QConvVoltage]
  ModulatorTimes/5(MPCC_u8ModulationSector) -> Scope/1, [MPCC_u8ModulationSector]
  [MPCC_f32MinSector] -> ModulatorTimes/9(MPCC_f32MinSector)
  [MPCC_f32Duty_Sector2] -> ModulatorTimes/4(MPCC_f32Duty_Sector2)
  [MPCC_f32Duty_Sector5] -> ModulatorTimes/7(MPCC_f32Duty_Sector5)
  [MPCC_f32Duty_Sector4] -> ModulatorTimes/6(MPCC_f32Duty_Sector4)
  [PI_f32DCLinkVoltage] -> ModulatorTimes/2(MPCC_f32DCLinkVoltage)
  ModulatorTimes/3(MPCC_f32Time2) -> [MPCC_f32Time2]
  [MPCC_f32Duty_Sector3] -> ModulatorTimes/5(MPCC_f32Duty_Sector3)
  Demux/1 -> [D], Delay/1
  Cast To Single6/1 -> [PI_f32DGridVoltage]
  Square1/1 -> Subtract/2
  Signal Copy/1 -> Square/1
  Subtract/1 -> Sqrt/1
  Square/1 -> Subtract/1
  Constant30/1 -> Divide4/2
  Divide4/1 -> Signal Copy/1
  From103/1 -> Divide4/1  "DClink"
  GridCurrentSecondPrediction/2(MPCC_f32MinSector) -> Cast To Single/1
  [PI_f32DCLinkVoltage] -> VoltageReferenceCalculation/16(MPCC_f32DCLinkVoltage)
  PI_f32DCLinkVoltageref/1 -> [PI_f32DCLinkVoltageref]
  Width/1 -> Data/2(Data_width), Start/2(Data_width), End/2(Data_width)
  Start/1(Data_out) -> Merge/1
  Constant3/1 -> Add/2, Add3/2
  Data/2(Iteration) -> Merge1/3
  Bus Selector1/2 -> Add3/1  "<signal2>"
  Merge/1 -> Mux/1  "SCI_Tx_Data"
  Data/1(Data_out) -> Merge/3
  Add3/1 -> Gain7/1
  Gain7/1 -> Mux1/2
  Counter Limited/1 -> If/1
  Mux/1 -> CodeGeneration/1(Input)
  Data_Conditioning/1(Out1) -> Width/1, Start/1(Data), End/1(Data), Data/1(Data)
  If/3 -> Data/Action
  If/2 -> End/Action
  Mux1/1 -> Data_Conditioning/1(In1)
  Add/1 -> Gain6/1
  Bus Selector1/1 -> Add/1  "<signal1>"
  Bus Creator/1 -> Bus Selector1/1
  End/2(Iteration) -> Merge1/2
  End/1(Data_out) -> Merge/2
  Merge1/1 -> Mux/2  "SCI_Tx_Iteration"
  If/1 -> Start/Action
  Start/2(Iteration) -> Merge1/1
  Gain6/1 -> Mux1/1
  Cast To Boolean/1 -> Subsystem1/Enable
  Cast To Single9/1 -> Subsystem1/1(In1)
  Cast To Single10/1 -> Subsystem1/2(In2)
  From124/1 -> Cast To Single10/1
  From123/1 -> Cast To Single9/1
  Constant36/1 -> Cast To Boolean/1
  Constant37/1 -> Subsystem2/Enable
  From128/1 -> Subsystem2/1(In1)
  From129/1 -> Subsystem2/2(In2)
  [PI_f32DGridCurrent] -> Signal Copy1/1
  Signal Copy1/1 -> Out1/1
  Demux/2 -> [Q], Delay1/1
  Gain2/1 -> Product/2  "Iau"
  Gain3/1 -> Product1/2  "Ibu"
  Gain4/1 -> Product2/2  "Icu"
  Product2/1 -> ?
  Constant51/1 -> Product2/1, Product1/1, Product/1
  MPCC_f32GridCurrentC/1 -> Gain20/1
  Gain20/1 -> Gain21/1  "Iau"
  Gain21/1 -> [PI_f32GridCurrentC]  "Iau"
  [PI_f32QGridVoltage] -> GridCurrentFirstPrediction/7(MPCC_f32QGridVoltage)
  [PI_f32DGridVoltage] -> GridCurrentFirstPrediction/6(MPCC_f32DGridVoltage)
  Gain23/1 -> Demux/1
  [D] -> dq_abc1/2(vd)
  [Q] -> dq_abc1/3(vq)
  [MPCC_f32ElectricalAngle_K_1] -> dq_abc1/1(theta)
  dq_abc1/2(Ib) -> Mux4/2
  dq_abc1/3(Ic) -> Mux4/3
  dq_abc1/1(Ia) -> Mux4/1
  [PI_f32DCLinkVoltage] -> SVM/2(Vdc)
  SVM/1(Dabc) -> Demux1/1
  Demux1/1 -> [PWM1_Duty]
  Demux1/2 -> [PWM2_Duty]
  Demux1/3 -> [PWM3_Duty]
  Constant48/1 -> Mux6/3
  Mux6/1 -> Alpha-Beta-Zero to dq0/1, Alpha-Beta-Zero to abc/1
  [D] -> Mux6/1
  [Q] -> Mux6/2
  Alpha-Beta-Zero to abc/1 -> SVM/1(Vabc)
  [MPCC_f32ElectricalAngle_K_1] -> AlphaBetaVoltageReferenceCalculation/3(MPCC_f32ElectricalAngle_K_1)
  [FG] -> AlphaBetaVoltageReferenceCalculation/1(MPCC_f32DVoltageReference)
  VoltageReferenceCalculation/1(MPCC_f32DVoltageReference) -> [MPCC_f32DVoltageReference]
  VoltageReferenceCalculation/2(MPCC_f32QVoltageReference) -> [MPCC_f32QVoltageReference]
  [MPCC_f32DConvVoltage] -> GridCurrentFirstPrediction/8(MPCC_f32DConvVoltage)
  [MPCC_f32QConvVoltage] -> GridCurrentFirstPrediction/9(MPCC_f32QConvVoltage)
  AlphaBetaVoltageReferenceCalculation/1(MPCC_f32AlphaVoltageReference) -> [PI_f32DGridCurrentReference]
  AlphaBetaVoltageReferenceCalculation/2(MPCC_f32BetaVoltageReference) -> [PI_f32QGridCurrentReference]
  [MPCC_f32ElectricalAngle] -> Alpha-Beta-Zero to dq0/2
  Alpha-Beta-Zero to dq0/1 -> Demux2/1
  Demux2/1 -> Square2/1
  Demux2/2 -> Square3/1
  Square2/1 -> Add10/1
  Square3/1 -> Add10/2
  Add10/1 -> Sqrt1/1
  Constant11/1 -> GridCurrentSecondPrediction/21(MPCC_f32QGridCurrent1), GridCurrentSecondPrediction/20(MPCC_f32DGridCurrent1)
  Constant18/1 -> Gain12/1
  [MPCC_f32AngularFrequency] -> VoltageReferenceCalculation/4(MPCC_f32AngularFrequency)
  Product1/1 -> [PI_f32GridCurrentB]  "Iau"
  Product/1 -> [PI_f32GridCurrentA]
  Constant25/1 -> Subsystem/4(Trip)
  [PWM2_Duty] -> Subsystem/2(PWM2)
  [PWM1_Duty] -> Subsystem/1(PWM1)
  [PWM3_Duty] -> Subsystem/3(PWM3)
  PI_f32DGridCurrentReference/1 -> [FG]
  MPCC_f32AngularFrequency/1 -> [MPCC_f32AngularFrequency]
  Cast To Single1/1 -> [PI_f32DGridCurrent]
  Cast To Single2/1 -> [PI_f32QGridCurrent]
  Cast To Single3/1 -> [PI_f32QGridVoltage]
  Sqrt1/1 -> Terminator/1
  [MPCC_f32AngularFrequency] -> ABCtoDQO/8(MPCC_f32AngularFrequency)
  ABCtoDQO/7(PI_f32DGridVoltage1) -> [MPCC_f32DGridVoltage_K_1]
  ABCtoDQO/8(PI_f32QGridVoltage1) -> [MPCC_f32QGridVoltage_K_1]
  [PI_f32QGridVoltage] -> GridCurrentSecondPrediction/10(MPCC_f32QGridVoltage)
  [PI_f32DGridVoltage] -> GridCurrentSecondPrediction/9(MPCC_f32DGridVoltage)
  [PI_f32DGridVoltage] -> VoltageReferenceCalculation/9(MPCC_f32DGridVoltage)
  [PI_f32QGridVoltage] -> VoltageReferenceCalculation/10(MPCC_f32QGridVoltage)
  [PI_f32DGridCurrent] -> VoltageReferenceCalculation/5(MPCC_f32DGridCurrent)
  [PI_f32QGridCurrent] -> VoltageReferenceCalculation/6(MPCC_f32QGridCurrent)
  [PI_f32QGridCurrent] -> GridCurrentSecondPrediction/19(MPCC_f32QGridCurrent)
  [PI_f32DGridCurrent] -> GridCurrentSecondPrediction/18(MPCC_f32DGridCurrent)
  From7/1 -> SOGI 1st/2(Vαβ)
  From10/1 -> SOGI 1st/1(w)
  SOGI 1st/2(qv) -> Bus Creator/2
  SOGI 1st/1(v) -> Bus Creator/1
  Constant16/1 -> Add4/2, Add5/2
  Start1/2(Iteration) -> Merge3/1
  Data1/2(Iteration) -> Merge3/3
  Data1/1(Data_out) -> Merge2/3
  If1/2 -> End1/Action
  Data_Conditioning1/1(Out1) -> Width1/1, Start1/1(Data), End1/1(Data), Data1/1(Data)
  Gain8/1 -> Mux3/1
  Start1/1(Data_out) -> Merge2/1
  Add5/1 -> Gain10/1
  Counter Limited1/1 -> If1/1
  Mux2/1 -> CodeGeneration1/1(Input)
  Bus Creator1/1 -> Bus Selector2/1
  Width1/1 -> Data1/2(Data_width), Start1/2(Data_width), End1/2(Data_width)
  End1/1(Data_out) -> Merge2/2
  If1/1 -> Start1/Action
  End1/2(Iteration) -> Merge3/2
  Bus Selector2/2 -> Add5/1  "<signal2>"
  Merge3/1 -> Mux2/2  "SCI_Tx_Iteration"
  Mux3/1 -> Data_Conditioning1/1(In1)
  Add4/1 -> Gain8/1
  Bus Selector2/1 -> Add4/1  "<signal1>"
  Merge2/1 -> Mux2/1  "SCI_Tx_Data"
  If1/3 -> Data1/Action
  Gain10/1 -> Mux3/2
  [PI_f32DGridCurrent] -> Subsystem6/1(In1)
  [PI_f32QGridCurrent] -> Subsystem6/2(In2)
  [MPCC_f32ElectricalAngle] -> Subsystem6/3(theta)
  Subsystem6/2(Iq) -> Bus Creator1/2
  Subsystem6/1(Id) -> Bus Creator1/1
  Cast To Single/1 -> [MPCC_f32MinSector]
  Gain11/1 -> VoltageReferenceCalculation/1(MPCC_f32RGrid)
  Gain12/1 -> VoltageReferenceCalculation/2(MPCC_f32LGrid)

== system Copy_of_AB_Final_of_MPC_Bandwidth_Result/Subsystem2 ==
  function : TriggerPort  TriggerType=function-call  VariantControl=(inherit)
  Constant : Constant  Value=boolean(1)
  Digital Output : c2837xDlib/Digital Output  GPIO_Number=GPIO8~GPIO15  GPIO_Bit0=off  GPIO_BIT0_Toggle=off  GPIO_Bit1=off  GPIO_BIT1_Toggle=off  GPIO_Bit2=off  GPIO_BIT2_Toggle=off  GPIO_Bit3=off  GPIO_BIT3_Toggle=off  GPIO_Bit4=off  GPIO_BIT4_Toggle=off  GPIO_Bit5=off  GPIO_BIT5_Toggle=off  GPIO_Bit6=on  GPIO_BIT6_Toggle=off  GPIO_Bit7=off  GPIO_BIT7_Toggle=off
  wires:
  Constant/1 -> Digital Output/1

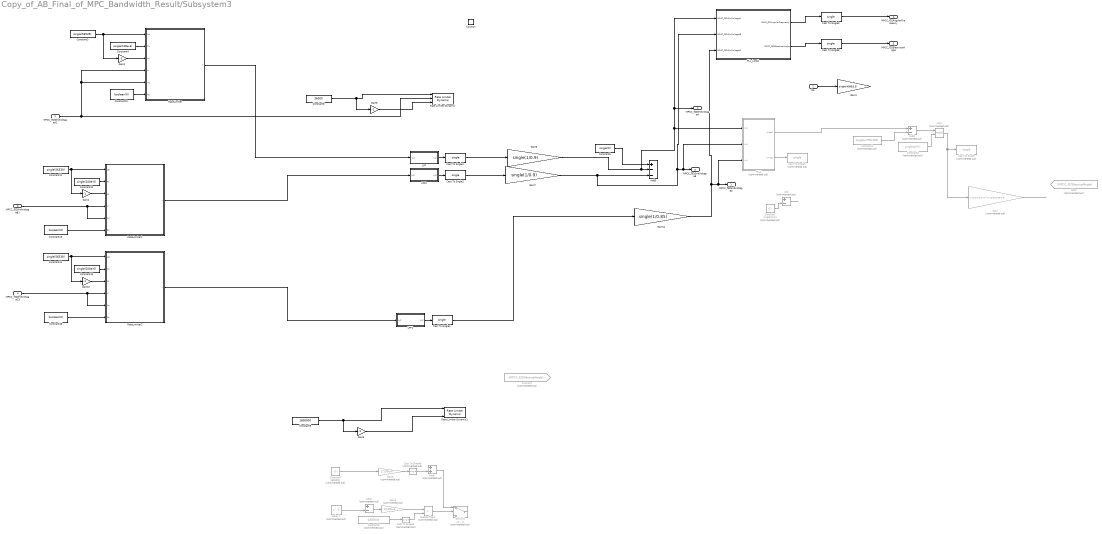
== system Copy_of_AB_Final_of_MPC_Bandwidth_Result/Subsystem3 ==
  MPCC_f32GridVoltageA2 : Inport
  Da : Inport  Port=2
  MPCC_f32GridVoltageB1 : Inport  Port=3
  MPCC_f32GridVoltageC3 : Inport  Port=4
  function : TriggerPort  TriggerType=function-call  VariantControl=(inherit)
  Add : Sum  Commented=on  Inputs=+-
  Add1 : Sum  Commented=on  Inputs=+-
  Add4 : Sum  Commented=on  Inputs=+-
  Add5 : Sum  Inputs=+--
  Add6 : Sum  Commented=on
  Cast To Single{,5..7} (4 alike) : DataTypeConversion  Commented=on  OutDataTypeStr=single  SaturateOnIntegerOverflow=off  RndMeth=Floor
  Cast To Single{1..4,8} (5 alike) : DataTypeConversion  OutDataTypeStr=single  SaturateOnIntegerOverflow=off  RndMeth=Floor
  Constant : Constant  Commented=on  Value=single(2*pi)
  Constant1 : Constant  Commented=on  Value=single(pi*90/180)
  Constant10 : Constant  Value=boolean(0)
  Constant11 : Constant  Value=single(56539)
  Constant12 : Constant  Value=single(100e-6)
  Constant13 : Constant  Value=boolean(0)
  Constant14 : Constant  Value=single(56539)
  Constant15 : Constant  Value=single(100e-6)
  Constant16 : Constant  Value=boolean(0)
  Constant2 : Constant  Commented=on  Value=single(pi*2)
  Constant3 : Constant  Value=single(56539)
  Constant4 : Constant  Value=single(100e-6)
  Constant5 : Constant  Value=single(0)
  Constant6 : Constant  Commented=on  Value=1800000
  Constant7 : Constant  Commented=on  Value=1800000
  Constant8 : Constant  Value=36000
  Constant9 : Constant  Value=1800000
  Delay1 : Delay  Commented=on  DelayLength=1  InitialConditionSource=Input port
      settings: InputPortMap=u0,p4
  From127 : From  Commented=on  GotoTag=MPCC_f32ElectricalAngle
  Gain : Gain  Commented=on  Gain=single(3.3/(2*pi))*single(4095/3.3)
  Gain1 : Gain  Gain=single(4095/3.3)
  Gain{2,4,8..10} (5 alike) : Gain  Gain=-1
  Gain11 : Gain  Gain=single(1/0.85)
  Gain3 : Gain  Commented=on  Gain=1/100e-6
  Gain5 : Gain  Commented=on  Gain=1/100e-6
  Gain6 : Gain  Gain=single(1/0.9)
  Gain7 : Gain  Gain=single(1/0.9)
  Goto : Goto  Commented=on  GotoTag=MPCC_f32ElectricalAngle
  GreaterThan1 : RelationalOperator  Commented=on  Operator=>  OutDataTypeStr=boolean  RndMeth=Simplest  InputSameDT=off
  LPF : Subsystem
  LPF1 : Subsystem
  LPF2 : Subsystem
  Mod : Math  Commented=on  Operator=mod
  PLL2 : Subsystem  Commented=on
  PLL_Loop1 : Subsystem
  Rate Limiter Dynamic : simulink/Discontinuities/Rate Limiter Dynamic
  Rate Limiter Dynamic1 : simulink/Discontinuities/Rate Limiter Dynamic
  RateLimiter : Subsystem
  RateLimiter1 : Subsystem
  RateLimiter2 : Subsystem
  Switch1 : Switch  Commented=on  Criteria=u2 > Threshold  SaturateOnIntegerOverflow=off  InputSameDT=off
  MPCC_f32GridVoltageC : Outport
  MPCC_f32GridVoltageA : Outport  Port=2
  MPCC_f32GridVoltageB : Outport  Port=3
  MPCC_f32AngularFrequency : Outport  Port=4
  MPCC_f32ElectricalAngle : Outport  Port=5
  wires:
  Cast To Single1/1 -> Gain6/1
  Constant5/1 -> Add5/1
  Cast To Single2/1 -> Gain7/1
  Constant/1 -> Add/2
  Add/1 -> ?
  Constant2/1 -> Mod/2
  PLL2/1(theta1) -> Add1/1
  Constant1/1 -> Add1/2
  Add1/1 -> Mod/1
  Da/1 -> Gain1/1
  LPF/1(y_k) -> Cast To Single1/1
  LPF2/1(y_k) -> Cast To Single2/1
  Gain/1 -> ?
  Gain7/1 -> Add5/3, PLL_Loop1/2(MPCC_f32GridVoltageB), PLL2/2(vb1), MPCC_f32GridVoltageB/1
  Delay1/1 -> Add4/2
  Add6/1 -> Switch1/1
  Constant7/1 -> Gain5/1
  GreaterThan1/1 -> Switch1/2
  Add4/1 -> Gain3/1
  Gain5/1 -> Cast To Single6/1
  Constant6/1 -> Cast To Single5/1
  Cast To Single5/1 -> GreaterThan1/2
  Cast To Single6/1 -> Add6/2
  Gain3/1 -> GreaterThan1/1
  MPCC_f32GridVoltageA2/1 -> RateLimiter/5(Xo), RateLimiter/4(U), Rate Limiter Dynamic/2
  Constant8/1 -> Gain8/1, Rate Limiter Dynamic/1
  Gain8/1 -> Rate Limiter Dynamic/3
  Constant9/1 -> Rate Limiter Dynamic1/1, Gain9/1
  Gain9/1 -> Rate Limiter Dynamic1/3
  Constant3/1 -> Gain2/1, RateLimiter/1(Up)
  Gain2/1 -> RateLimiter/3(Lo)
  Constant4/1 -> RateLimiter/2(Ts)
  Constant10/1 -> RateLimiter/6(Rs)
  RateLimiter/1(Y) -> LPF/1(u_k)
  Constant11/1 -> Gain4/1, RateLimiter1/1(Up)
  Constant12/1 -> RateLimiter1/2(Ts)
  Gain4/1 -> RateLimiter1/3(Lo)
  MPCC_f32GridVoltageB1/1 -> RateLimiter1/5(Xo), RateLimiter1/4(U)
  Constant13/1 -> RateLimiter1/6(Rs)
  RateLimiter1/1(Y) -> LPF2/1(u_k)
  RateLimiter2/1(Y) -> LPF1/1(u_k)
  Constant16/1 -> RateLimiter2/6(Rs)
  Gain10/1 -> RateLimiter2/3(Lo)
  Constant15/1 -> RateLimiter2/2(Ts)
  Constant14/1 -> Gain10/1, RateLimiter2/1(Up)
  LPF1/1(y_k) -> Cast To Single4/1
  Cast To Single4/1 -> Gain11/1
  MPCC_f32GridVoltageC3/1 -> RateLimiter2/5(Xo), RateLimiter2/4(U)
  Gain11/1 -> PLL_Loop1/3(MPCC_f32GridVoltageC), PLL2/3(vc1), MPCC_f32GridVoltageC/1
  Gain6/1 -> PLL_Loop1/1(MPCC_f32GridVoltageA), MPCC_f32GridVoltageA/1, PLL2/1(va1), Add5/2
  Mod/1 -> Gain/1, Cast To Single/1
  PLL2/2(omega) -> Cast To Single7/1
  PLL_Loop1/1(MPCC_f32AngularFrequency) -> Cast To Single3/1
  PLL_Loop1/2(MPCC_f32ElectricalAngle) -> Cast To Single8/1
  Cast To Single3/1 -> MPCC_f32AngularFrequency/1
  Cast To Single8/1 -> MPCC_f32ElectricalAngle/1

== system Copy_of_AB_Final_of_MPC_Bandwidth_Result/Subsystem4 ==
  function : TriggerPort  TriggerType=function-call  VariantControl=(inherit)
  Constant : Constant  Value=boolean(0)
  Digital Output : c2837xDlib/Digital Output  GPIO_Number=GPIO8~GPIO15  GPIO_Bit0=off  GPIO_BIT0_Toggle=off  GPIO_Bit1=off  GPIO_BIT1_Toggle=off  GPIO_Bit2=off  GPIO_BIT2_Toggle=off  GPIO_Bit3=off  GPIO_BIT3_Toggle=off  GPIO_Bit4=off  GPIO_BIT4_Toggle=off  GPIO_Bit5=off  GPIO_BIT5_Toggle=off  GPIO_Bit6=on  GPIO_BIT6_Toggle=off  GPIO_Bit7=off  GPIO_BIT7_Toggle=off
  wires:
  Constant/1 -> Digital Output/1
